simulink model "f"  (R2023a)
settings: Solver=ode1  StartTime=0.0  StopTime=15.0  RelTol=1e-3
settings Model: Creator=eriknymobohne  LastModifiedBy=eriknymobohne

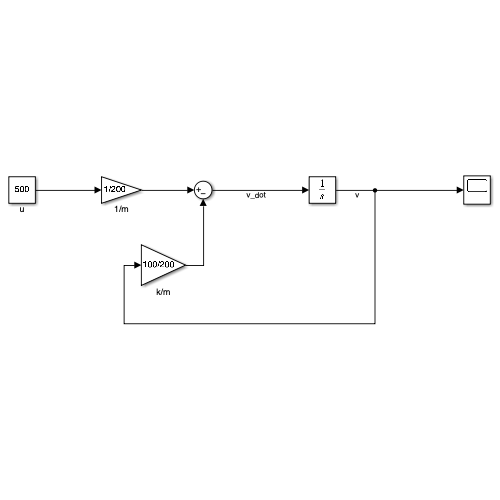
[thumbnail: Simulink's stored preview of the top-level diagram]
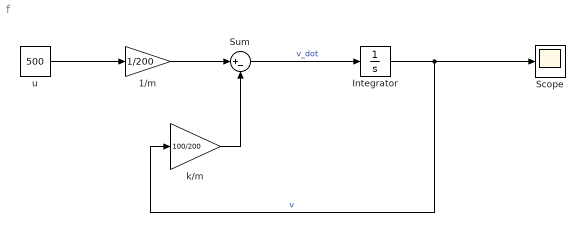
== system f ==
  1/m : Gain  Gain=1/200
  Integrator : Integrator
  Scope : Scope
  Sum : Sum  Inputs=|+-
  k/m : Gain  Gain=100/200
  u : Constant  Value=500
  wires:
  Sum/1 -> Integrator/1  "v_dot"
  Integrator/1 -> k/m/1, Scope/1  "v"
  k/m/1 -> Sum/2
  1/m/1 -> Sum/1
  u/1 -> 1/m/1
